simulink model "ex_blkCornerDetection_edited"  (R2023b)
settings: Solver=FixedStepDiscrete  StartTime=0.0  StopTime=0  RelTol=1e-3
undefined symbols (not defined in the file or in its folder): gray, Rec, SDTV
libraries: visiontextngfix x2, visionconversions x1, dspinverses x1, dspmathops x1, visionsources x1
settings Model: Creator=The MathWorks, Inc.  LastModifiedBy=Alyssa
settings DebuggingCC: ParameterPrecisionLossMsg=none  UnconnectedInputMsg=warning  UnconnectedOutputMsg=warning  UnconnectedLineMsg=warning  IntegerSaturationMsg=none
settings ModelReferenceCC: EnableRefExpFcnMdlSchedulingChecks=on
settings RTWCC: DLArmComputeVersion=19.05

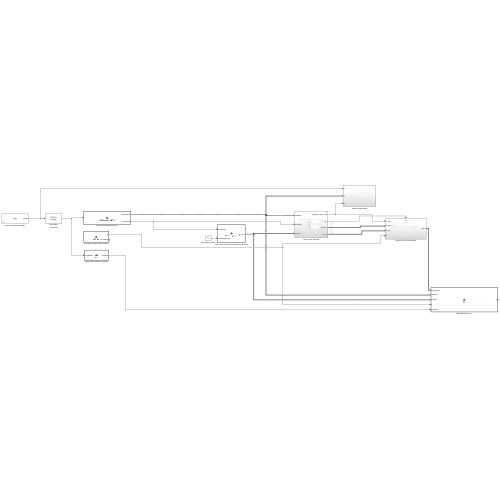
[thumbnail: Simulink's stored preview of the top-level diagram]
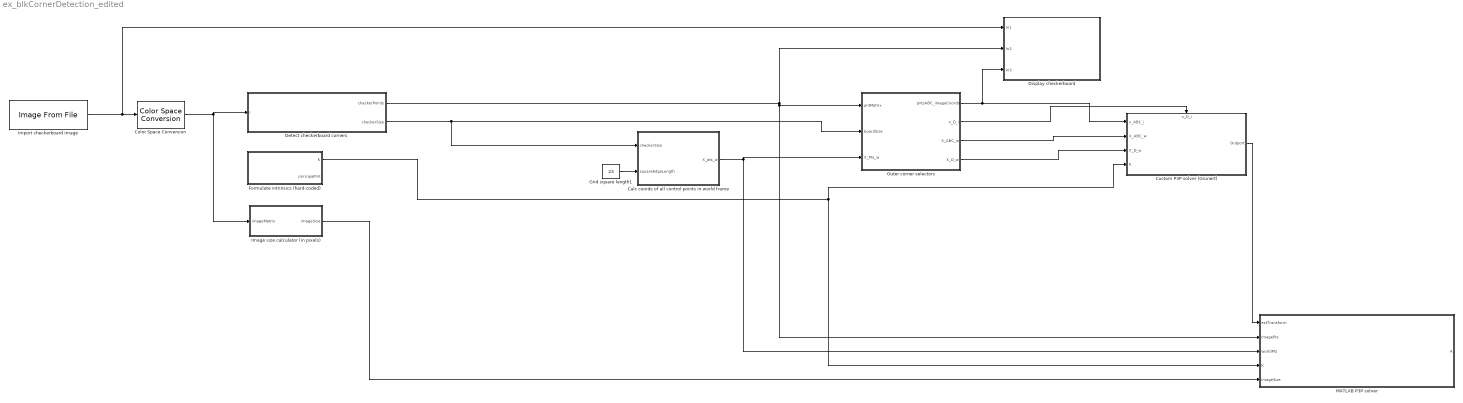
== system ex_blkCornerDetection_edited ==
  Calc coords of all control points in world frame : MATLAB Function  TreatAsAtomicUnit=on
  Color Space Conversion : visionconversions/Color Space  Conversion  conversion=Obsolete  conversionActive=R'G'B' to intensity  wp_str=D65  rec=Rec. 601 (SDTV)  sys=1125/60/2:1  imagePorts=One multidimensional signal
  Custom P3P solver (Grunert) : Subsystem
      settings: PortSchema="{\"entries\":[{\"content\":{\"sides\":[{\"content\":{\"connectorIds\":[\"In1\",\"In2\",\"In3\",\"In4\"]},\"type\":\"ConnectorPlacement.EquallySpacedRectSide\",\"uuid\":\"ab8d8f47-a078-4904-b229-676f132fd238\"},{\"content\":{\"connectorIds\":[\"Out1\"],\"side\":\"RIGHT\"},\"type\":\"ConnectorPlacement.EquallySpacedRectSide\",\"uuid\":\"00cb969a-2808-4efa-a104-ddec5f07b100\"},{\"content\":{\"connectorIds\":[\"In5\"],\"side\":\"TOP\"},\"type\":\"ConnectorPlacement.EquallySpacedRectSide\",\"uuid\":\"2fc50beb-0e06-41d1-87ca-520f8001ed43\"}]},\"type\":\"ConnectorPlacement.EquallySpacedConnector\",\"uuid\":\"61196fa6-a691-4b7f-8fee-5a47d7d03c1d\"}],\"packageUris\":[\"http://schema.mathworks.com/mf0/Connector/R2020b\"],\"version\":\"1.0\"}"
  Detect checkerboard corners : MATLAB Function  TreatAsAtomicUnit=on
  Display checkerboard : Subsystem
  Formulate intrinsics (hard-coded) : MATLAB Function  TreatAsAtomicUnit=on
  Grid square length1 : Constant  Value=23
  Image size calculator (in pixels) : MATLAB Function  TreatAsAtomicUnit=on
  Import checkerboard image : visionsources/Image From File  Tag=vipblks_nd  FileName=C:\Users\Alyssa\OneDrive - University of Cape Town\Vision\ESP32-CAM\CamCalibrationPics\8.jpg  Ts=inf  imagePorts=One multidimensional signal  OutPortLabels=R|G|B  ImageDataType=Inherit from input image  sdImageDataType=uint(8)  Signed=on  WordLength=16  FractionLengthMode=User-defined  FractionLength=15
  MATLAB P3P solver : MATLAB Function  TreatAsAtomicUnit=on
  Outer corner selectors : Subsystem
  wires:
  Color Space Conversion/1 -> Image size calculator (in pixels)/1(imageMatrix), Detect checkerboard corners/1(I)
  Import checkerboard image/1 -> Display checkerboard/1(In1), Color Space Conversion/1
  Detect checkerboard corners/2(checkerSize) -> Calc coords of all control points in world frame/1(checkerSize), Outer corner selectors/2(boardSize)
  Formulate intrinsics (hard-coded)/1(K) -> Custom P3P solver (Grunert)/4(K), MATLAB P3P solver/4(K)
  Custom P3P solver (Grunert)/1(Outport) -> MATLAB P3P solver/1(estTransform)
  Calc coords of all control points in world frame/1(X_pts_w) -> MATLAB P3P solver/3(worldPts), Outer corner selectors/3(X_Pts_w)
  Grid square length1/1 -> Calc coords of all control points in world frame/2(squareEdgeLength)
  Outer corner selectors/1(pntsABC_imageCoords) -> Custom P3P solver (Grunert)/1(x_ABC_i), Display checkerboard/3(In3)
  Outer corner selectors/2(x_D_i) -> Custom P3P solver (Grunert)/5(x_D_i)
  Outer corner selectors/3(X_ABC_w) -> Custom P3P solver (Grunert)/2(X_ABC_w)
  Outer corner selectors/4(X_D_w) -> Custom P3P solver (Grunert)/3(X_D_w)
  Detect checkerboard corners/1(checkerPoints) -> MATLAB P3P solver/2(imagePts), Outer corner selectors/1(pntMatrix), Display checkerboard/2(In2)
  Image size calculator (in pixels)/1(imageSize) -> MATLAB P3P solver/5(imageSize)

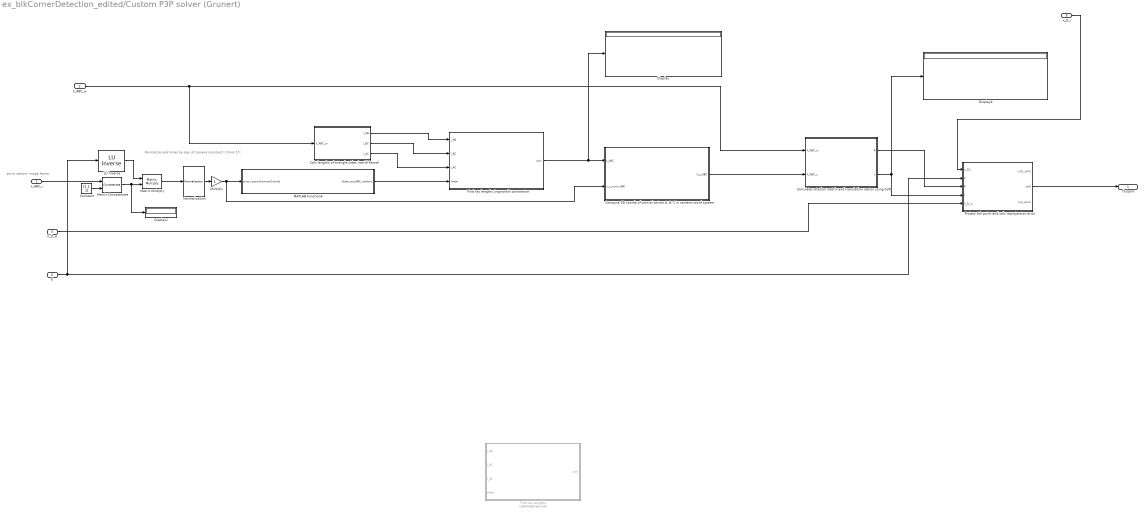
== system ex_blkCornerDetection_edited/Custom P3P solver (Grunert) ==
  note: point vectors image frame
  note: Normalize and times by sign of camera constant (I think 1?)
  x_ABC_i : Inport
  X_ABC_w : Inport  Port=2
  X_D_w : Inport  Port=3
  K : Inport  Port=4
  x_D_i : Inport  Port=5
  " LU Inverse" : dspinverses/ LU Inverse
  Calc lengths of triangle sides (world frame) : MATLAB Function  TreatAsAtomicUnit=on
  Calculate rotation matrix and translation vector using SVD : MATLAB Function  TreatAsAtomicUnit=on
  "Compute 3D coords of control points A, B, C in camera coord system" : MATLAB Function  TreatAsAtomicUnit=on
  Constant : Constant  Value=[1 1 1]  VectorParams1D=off
  Display : Display
  Display1 : Display
  Display4 : Display
  Find ray lengths : MATLAB Function  Commented=on  TreatAsAtomicUnit=on
  Find ray lengths jingnanshi convention : MATLAB Function  TreatAsAtomicUnit=on
  MATLAB Function4 : MATLAB Function  TreatAsAtomicUnit=on
  Matrix Concatenate : Concatenate  Mode=Multidimensional array
  Matrix Multiply : Product  Multiplication=Matrix(*)
  Multiply : Gain
  Normalization : dspmathops/Normalization  NormType=2-norm  Bias=1e-10  NormOver=Each column  Dimension=1  roundingMode=Floor  overflowMode=off  accumDataTypeStr=Inherit: Same as product output  accumLastDataTypeStr=Inherit: Same as product output  outputDataTypeStr=Inherit: Same as product output  outputMin=[]  outputMax=[]  outputLastDataTypeStr=Inherit: Same as product output
  Project 4th point and calc reprojection error : MATLAB Function  TreatAsAtomicUnit=on
  Outport : Outport
  wires:
  Calculate rotation matrix and translation vector using SVD/1(R) -> Project 4th point and calc reprojection error/3(R)
  Multiply/1 -> "Compute 3D coords of control points A, B, C in camera coord system"/2(x_c_norm_ABC), MATLAB Function4/1(pnts_vectorsCameraCoords)
  Normalization/1 -> Multiply/1
  MATLAB Function4/1(theta_raysABC_radians) -> Find ray lengths jingnanshi convention/4(theta)
  "Compute 3D coords of control points A, B, C in camera coord system"/1(X_c_ABC) -> Calculate rotation matrix and translation vector using SVD/2(X_ABC_c)
  Calculate rotation matrix and translation vector using SVD/2(t) -> Project 4th point and calc reprojection error/4(t), Display4/1
  X_D_w/1 -> Project 4th point and calc reprojection error/5(X_D_w)
  X_ABC_w/1 -> Calc lengths of triangle sides (world frame)/1(X_ABC_w), Calculate rotation matrix and translation vector using SVD/1(X_ABC_w)
  Calc lengths of triangle sides (world frame)/3(l_AC) -> Find ray lengths jingnanshi convention/3(l_AC)
  Calc lengths of triangle sides (world frame)/1(l_AB) -> Find ray lengths jingnanshi convention/1(l_AB)
  Calc lengths of triangle sides (world frame)/2(l_BC) -> Find ray lengths jingnanshi convention/2(l_BC)
  K/1 -> " LU Inverse"/1, Project 4th point and calc reprojection error/2(K)
  x_D_i/1 -> Project 4th point and calc reprojection error/1(x_D_i)
  Project 4th point and calc reprojection error/2(soln) -> Outport/1
  Find ray lengths jingnanshi convention/1(soln) -> "Compute 3D coords of control points A, B, C in camera coord system"/1(s_ABC), Display/1
  x_ABC_i/1 -> Matrix Concatenate/1
  Matrix Concatenate/1 -> Display1/1, Matrix Multiply/2
  " LU Inverse"/1 -> Matrix Multiply/1
  Matrix Multiply/1 -> Normalization/1
  Constant/1 -> Matrix Concatenate/2

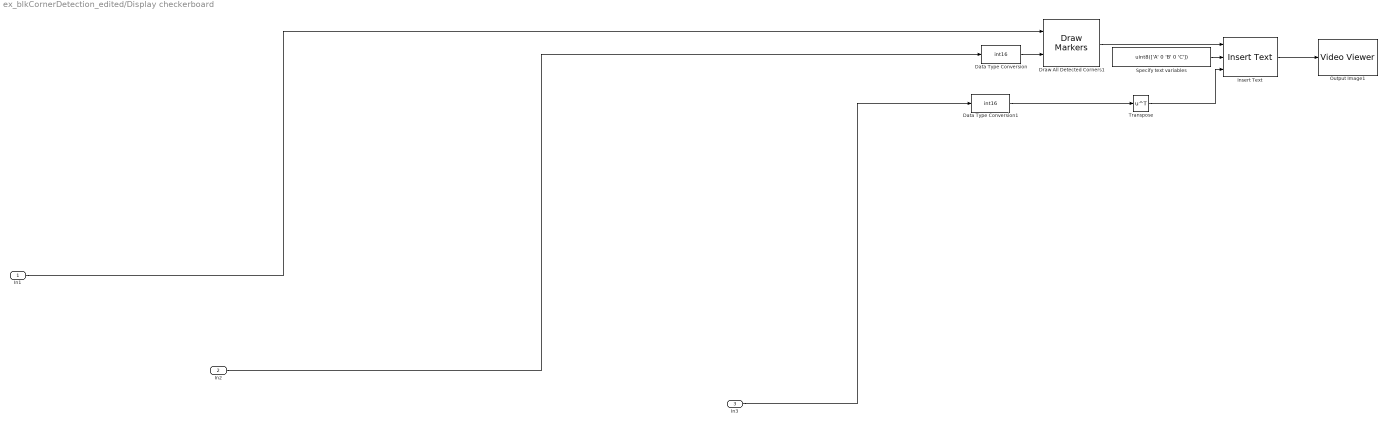
== system ex_blkCornerDetection_edited/Display checkerboard ==
  In1 : Inport
  In2 : Inport  Port=2
  In3 : Inport  Port=3
  Data Type Conversion : DataTypeConversion  OutDataTypeStr=int16  SaturateOnIntegerOverflow=off  RndMeth=Floor
  Data Type Conversion1 : DataTypeConversion  OutDataTypeStr=int16  SaturateOnIntegerOverflow=off  RndMeth=Floor
  Draw All Detected Corners1 : visiontextngfix/Draw Markers  shape=Circle  size=9  fill=on  fillClrSource=Specify via dialog  display=User-specified value  intensity=200  color=[250 0 0]  opacity=0.6  viewport=Entire image  antialiasing=off  inType=Obsolete  imagePorts=One multidimensional signal  roundingMode=Floor  overflowMode=off  memoryMode=Specify word length  memoryWordLength=16  memoryFracLength=15  prodOutputMode=Binary point scaling  prodOutputWordLength=32  prodOutputFracLength=14
  Insert Text : visiontextngfix/Insert Text  inputType=Obsolete  theText='%s'  getTextLocFrom=Input port  textLoc=[100 100]  getTextColorFrom=Specify via dialog  textColor=[0 255 0]  getTextIntensityFrom=Specify via dialog  textIntensity=1  getTextOpacityFrom=Specify via dialog  textOpacity=1.0  dummyVar2=0  dummyVar3=0  dummyVar4=0  imagePorts=One multidimensional signal  isInputTransposed=off  fontFace=LucidaSansRegular  dummyVar1=0  blockFontSize=60  antiAliased=on
  Output Image1 : VideoViewer  colormapValue=gray(256)  FigPos=[2113 930 833 715]
  Specify text variables : Constant  Value=uint8(['A' 0 'B' 0 'C'])
  Transpose : Math  Operator=transpose
  wires:
  Data Type Conversion/1 -> Draw All Detected Corners1/2
  Draw All Detected Corners1/1 -> Insert Text/1
  Specify text variables/1 -> Insert Text/2
  Transpose/1 -> Insert Text/3
  In1/1 -> Draw All Detected Corners1/1
  Insert Text/1 -> Output Image1/1
  Data Type Conversion1/1 -> Transpose/1
  In3/1 -> Data Type Conversion1/1
  In2/1 -> Data Type Conversion/1

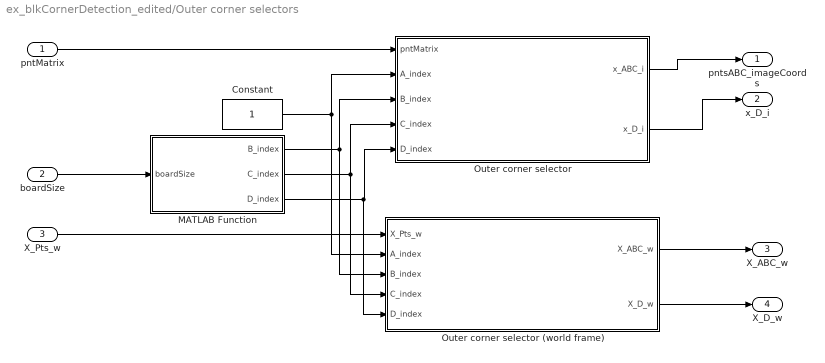
== system ex_blkCornerDetection_edited/Outer corner selectors ==
  pntMatrix : Inport
  boardSize : Inport  Port=2
  X_Pts_w : Inport  Port=3
  Constant : Constant
  MATLAB Function : MATLAB Function  TreatAsAtomicUnit=on
  Outer corner selector : MATLAB Function  TreatAsAtomicUnit=on
  Outer corner selector (world frame) : MATLAB Function  TreatAsAtomicUnit=on
  pntsABC_imageCoords : Outport
  x_D_i : Outport  Port=2
  X_ABC_w : Outport  Port=3
  X_D_w : Outport  Port=4
  wires:
  Outer corner selector/2(x_D_i) -> x_D_i/1
  Outer corner selector (world frame)/1(X_ABC_w) -> X_ABC_w/1
  Outer corner selector/1(x_ABC_i) -> pntsABC_imageCoords/1
  Outer corner selector (world frame)/2(X_D_w) -> X_D_w/1
  boardSize/1 -> MATLAB Function/1(boardSize)
  pntMatrix/1 -> Outer corner selector/1(pntMatrix)
  X_Pts_w/1 -> Outer corner selector (world frame)/1(X_Pts_w)
  Constant/1 -> Outer corner selector/2(A_index), Outer corner selector (world frame)/2(A_index)
  MATLAB Function/1(B_index) -> Outer corner selector/3(B_index), Outer corner selector (world frame)/3(B_index)
  MATLAB Function/2(C_index) -> Outer corner selector/4(C_index), Outer corner selector (world frame)/4(C_index)
  MATLAB Function/3(D_index) -> Outer corner selector (world frame)/5(D_index), Outer corner selector/5(D_index)

== matlab function ex_blkCornerDetection_edited/Custom P3P solver (Grunert)/Project 4th point and calc reprojection error ==
  data: x_D_i input; K input; R input; x_D_i_proj output size=[2,4]; t input; X_D_w input; soln output size=[3,4]; min_error output
function [x_D_i_proj, soln, min_error]= fcn(x_D_i, K, R, t, X_D_w)

%Calculate the projection of a fourth point onto the image plane, based on 
%the candidate rotation matrices and translation vectors. Later, we
%will check how well this corresponds with where it was actually observed.
    
    %Initialise vector
    x_D_i_proj = zeros(2,4); %where i stands for "image plane"
    x_D_i_proj_homo = zeros(3,4); %where i stands for "image plane"
    error = zeros(1,4);     %reprojection error
    soln = zeros(3, 4);

    %For each possible solution
    for n=1: size(R, 3)

        %Calculate projection of the point D
        x_D_i_proj_homo(:, n) = K * (  (R(:, :, n) * X_D_w)  + t(:,n)  );

        %Normalise by the 3rd dimension
        x_D_i_proj(1,n) = x_D_i_proj_homo(1,n)/x_D_i_proj_homo(3,n);
        x_D_i_proj(2,n) = x_D_i_proj_homo(2,n)/x_D_i_proj_homo(3,n);

        %Calculate reprojection error
        error(1, n) = norm(x_D_i - x_D_i_proj(:, n));
    
    end

    %Choose lower reprojection error
    error(1, 1) = norm(x_D_i - x_D_i_proj(:, 1));
    min_error = error(1,1);
    soln = [R(:, :, 1) t(:,1)];
    
    for j=2 : size(x_D_i_proj, 2)
        
        if error(1, j) < min_error
            min_error = error(1, j);
            soln = [R(:, :, j) t(:,j)]
        end
    
    end

== matlab function ex_blkCornerDetection_edited/MATLAB P3P solver ==
  data: estTransform input; imagePts input; worldPts input; K input; imageSize input; A output
function A = fcn(estTransform, imagePts, worldPts, K, imageSize)

    %imagePts_vert = transpose(imagePts);
    %worldPts_vert = transpose(worldPts);
    focalLngth = [K(1,1) K(2,2)];
    principalPnt = [K(1,3) K(2,3)];

    coder.extrinsic('builtinP3P');
    A = zeros(4,4);

    
    estTransform_R_inv = inv(estTransform(:, 1:3));
    estTransform_negTranslation_Rotated = estTransform_R_inv * (-estTransform(:, 4));

    A = builtinP3P(imagePts, worldPts, focalLngth, principalPnt, imageSize, estTransform_negTranslation_Rotated, estTransform_R_inv)

    %intr = cameraIntrinsics(focalLngth, principalPnt, imageSize)

    %worldPose = estworldpose(imagePts_vert, worldPts_vert, intr)

    %pcshow(worldPts,VerticalAxis="Y",VerticalAxisDir="down", ...
    %MarkerSize=30);
    %hold on
    %plotCamera(Size=10,Orientation=worldPose.R', ...
    %    Location=worldPose.Translation);
    %hold off

== matlab function ex_blkCornerDetection_edited/Image size calculator (in pixels) ==
  data: imageMatrix input; imageSize output
function imageSize = fcn(imageMatrix)

imageSize = [size(imageMatrix, 1) size(imageMatrix,2)];

== matlab function ex_blkCornerDetection_edited/Custom P3P solver (Grunert)/Find ray lengths jingnanshi convention ==
  data: l_AB input; soln output size=[4, 3]; l_BC input; l_AC input; theta input
function soln = fcn(l_AB, l_BC, l_AC, theta)

soln = zeros(4, 3);


%Calculate polynomial coefficients
a = l_AC;
b = l_BC;
c = l_AB;

gamma = theta(1); %theta_AB
alpha = theta(3); %theta_AC
beta = theta(2); %theta_BC


a2minc2ovb2 =  (a^2 - c^2) / b^2 ;
a2plusc2ovb2 =  (a^2 + c^2) / b^2; 


A0 = (1 + a2minc2ovb2)^2   -   4*((a*cos(gamma)/b)^2);
A1 = - a2minc2ovb2 * (1 + a2minc2ovb2) * cos(beta)     +    2 * ((a * cos(gamma) /  b)^2) * cos (beta)     -     (1 - a2plusc2ovb2) * cos(alpha) * cos(gamma);
A1 = 4 * A1;
A2 = a2minc2ovb2^2   -   1   +   2*((a2minc2ovb2 * cos(beta))^2)  +  2 *(  ((b^2 - c^2)/(b^2))  * (cos(alpha))^2  )   - 4*a2plusc2ovb2*cos(alpha)*cos(beta)*cos(gamma)   +   2*((b^2 - a^2)/(b^2))*((cos(gamma))^2);
A2 = 2* A2;
A3 = a2minc2ovb2 * (1 - a2minc2ovb2) * cos(beta)    -   (1 - a2plusc2ovb2) * cos(alpha) * cos(gamma)    +   2 * ((c * cos(alpha)/b)^2) * cos(beta);
A3 = 4 * A3;
A4 = (a2minc2ovb2 -1)^2   - (2 * c * cos(alpha) / b)^2;

%Solve polynomial
%instead of u and v for polynomial, use g and h - i.e., g = s2/s1 and h =
%s3/s1
p = [A4 A3 A2 A1 A0];
h = roots(p);
%choose only real roots - maybe this is not necessary?
h = h(imag(h)==0);
h = real(h);

%%%%%%%%%%%%%%%%%%%%%%%%%%%%%%%%%%%%%%%%%
%%%%%%%%%%%%%Find ray lengths

%For s1, which corresponds to sB. Should end up with 4 solns
%s_A =    (b^2) / (1 + h.^2  +  2*h*cos(beta)  )     ;
%s_A = s_A(s_A~=0);
%s_A = transpose(s_A);
%s_A = s_A.^0.5;


%Find s2, which corresponds to sC.
counter = 1
for i = 1:numel(h)

    s_1 = (b^2) / (1 + (h(i)^2) - 2*h(i)*cos(beta));
    s_1 = sqrt(s_1);

    G2 = s_1^2;
    G1 = - 2 * (s_1^2) * cos(gamma);
    G0 = (s_1^2 -c^2);

    g = roots([G2 G1 G0]);
    g = g(imag(g)==0);
    g = real(g);

    %First, solve for s_C, since it only depends on h and s_A:

    for j = 1:numel(g)
        soln(counter, 1) = s_1 * g(j);
        soln(counter, 3) = s_1 * h(i);
        soln(counter, 2) = s_1; 
        counter = counter +1
    end

end

== matlab function ex_blkCornerDetection_edited/Outer corner selectors/MATLAB Function ==
  data: boardSize input; B_index output; C_index output; D_index output
function [B_index, C_index, D_index]= fcn(boardSize)

B_index = boardSize(1) - 1;
C_index = ((boardSize(1) - 1) * (boardSize(2) - 2)) + 1;
D_index = ((boardSize(1) - 1) * (boardSize(2) - 1)) ;

== matlab function ex_blkCornerDetection_edited/Calc coords of all control points in world frame ==
  data: X_pts_w output size=[60, 3]; checkerSize input; squareEdgeLength input
function X_pts_w = calcPtoPLengths_world(checkerSize, squareEdgeLength)
    
    boardWidth = checkerSize(2);
    boardHeight = checkerSize(1);
    X_pts_w = zeros((boardWidth-1)*(boardHeight-1), 3)

    %for each column
    for c=1 : boardWidth-1
        for r = 1: boardHeight-1
            x = (c-1)*squareEdgeLength;
            y = (r-1)*squareEdgeLength;
            z = 0;
            X_pts_w(  (((c-1)*(boardHeight-1)) + r), 1) = x;
            X_pts_w(  (((c-1)*(boardHeight-1)) + r), 2) = y;
            X_pts_w(  (((c-1)*(boardHeight-1)) + r), 3) = z;
        end
    end

== matlab function ex_blkCornerDetection_edited/Custom P3P solver (Grunert)/Calc lengths of triangle sides (world frame) ==
  data: X_ABC_w input; l_AB output; l_BC output; l_AC output
function [l_AB, l_BC, l_AC]= fcn(X_ABC_w)

l_AB = norm(X_ABC_w(:,1)-X_ABC_w(:,2));
l_AC = norm(X_ABC_w(:,1)-X_ABC_w(:,3));
l_BC = norm(X_ABC_w(:,2)-X_ABC_w(:,3));

== matlab function ex_blkCornerDetection_edited/Detect checkerboard corners ==
  data: checkerPoints output size=[60, 2]; I input; checkerSize output size=[1, 2]
function [checkerPoints, checkerSize]= findCheckerboardPnts(I)

%I = imread(fullfile('C:\Users\Alyssa\OneDrive - University of Cape Town\Vision\ESP32-CAM\CamCalibrationPics', '1.jpg'));
Points = detectCheckerboardPoints(I);
[~,checkerSize] = detectCheckerboardPoints(I)
checkerPoints = round(Points);
%checkerSize = Size;
%checkerPoints = imagePoints;

== matlab function ex_blkCornerDetection_edited/Formulate intrinsics (hard-coded) ==
  data: K output; principalPnt output
function [K, principalPnt]= intrinsics

    fx = 1274.58238813250;
    fy = 1273.36371905619;
    Ox = 627.693937913345;
    Oy = 405.441250468717;

    K = [fx 0 Ox; 0 fy Oy; 0 0 1];

    principalPnt = [627.693937913345; 405.441250468717];

== matlab function ex_blkCornerDetection_edited/Outer corner selectors/Outer corner selector (world frame) ==
  data: X_Pts_w input; X_ABC_w output size=[3, 3]; X_D_w output size=[3, 1]; A_index input; B_index input; C_index input; D_index input
function [X_ABC_w, X_D_w]= calcPtoPLengths_world(X_Pts_w, A_index, B_index, C_index, D_index)
    
    X_A_w = X_Pts_w(A_index, :);
    X_B_w = X_Pts_w(B_index, :);
    X_C_w = X_Pts_w(C_index, :);
    X_D_w_vert = X_Pts_w(D_index, :);

    X_ABC_w_vert = [X_A_w; X_B_w; X_C_w];
    X_ABC_w = transpose(X_ABC_w_vert);
    X_D_w = transpose(X_D_w_vert);

== matlab function ex_blkCornerDetection_edited/Outer corner selectors/Outer corner selector ==
  data: x_ABC_i output; x_D_i output; pntMatrix input; A_index input; B_index input; C_index input; D_index input
function [x_ABC_i, x_D_i] = calcPntVectors_PrincipalPntToImagePlane(pntMatrix, A_index, B_index, C_index, D_index)

%Obtain pixel positions
A_u = pntMatrix(A_index,1);
A_v = pntMatrix(A_index,2);

B_u = pntMatrix(B_index, 1);
B_v = pntMatrix(B_index, 2);

C_u = pntMatrix( C_index , 1);
C_v = pntMatrix( C_index , 2);

D_u = pntMatrix( D_index, 1);
D_v = pntMatrix(D_index, 2);


%Created augmented U matrices - i.e., add extra row of "1"
x_ABC_i = [A_u B_u C_u; A_v B_v C_v]
%pnts_U_ABC_aug = [pnts_U_ABC; 1 1 1];

%pnts_X_c = inv(K) * pnts_U_ABC_aug;

%pntVectors_cameraCoords = pnts_X_c;
%pntsABC_imageCoords = pnts_U_ABC;
%pntsABCD_imageCoords = [A_u B_u C_u D_u; A_v B_v C_v D_v];
x_D_i = [D_u; D_v];

== matlab function ex_blkCornerDetection_edited/Custom P3P solver (Grunert)/MATLAB Function4 ==
  data: pnts_vectorsCameraCoords input; theta_raysABC_radians output
function theta_raysABC_radians = calcProjectionRayAngles(pnts_vectorsCameraCoords)

A_x_c = pnts_vectorsCameraCoords(:,1);
B_x_c = pnts_vectorsCameraCoords(:,2);
C_x_c = pnts_vectorsCameraCoords(:,3);

%theta_AB = acos(dot(A_x_c, B_x_c));
%theta_BC = acos(dot(B_x_c, C_x_c));
%theta_AC = acos(dot(C_x_c, A_x_c));

%theta_AB = atan2(norm(cross(A_x_c, B_x_c)), dot(A_x_c, B_x_c));
%theta_BC = atan2(norm(cross(B_x_c, C_x_c)), dot(B_x_c, C_x_c));
%theta_AC = atan2(norm(cross(A_x_c, C_x_c)), dot(A_x_c, C_x_c)); 

theta_AB = acos(dot(A_x_c, B_x_c)/(norm(A_x_c)*norm(B_x_c)));
theta_BC = acos(dot(B_x_c, C_x_c)/(norm(B_x_c)*norm(C_x_c)));
theta_AC = acos(dot(A_x_c, C_x_c)/(norm(A_x_c)*norm(C_x_c)));


theta_raysABC_radians = [theta_AB; theta_BC; theta_AC];

== matlab function ex_blkCornerDetection_edited/Custom P3P solver (Grunert)/Find ray lengths ==
  data: l_AB input; soln output size=[4, 3]; l_BC input; l_AC input; theta input
function soln = fcn(l_AB, l_BC, l_AC, theta)

soln = zeros(4, 3);


%Calculate polynomial coefficients
a = l_BC;
b = l_AC;
c = l_AB;

gamma = theta(3); %theta_AC
alpha = theta(2); %theta_BC
beta = theta(1); %theta_AB


a2minc2ovb2 =  (a^2 - c^2) / b^2 ;
a2plusc2ovb2 =  (a^2 + c^2) / b^2; 


A0 = (1 + a2minc2ovb2)^2   -   4*((a*cos(gamma)/b)^2);
A1 = - a2minc2ovb2 * (1 + a2minc2ovb2) * cos(beta)     +    2 * ((a * cos(gamma) /  b)^2) * cos (beta)     -     (1 - a2plusc2ovb2) * cos(alpha) * cos(gamma);
A1 = 4 * A1;
A2 = a2minc2ovb2^2   -   1   +   2*((a2minc2ovb2 * cos(beta))^2)  +  2 *(  ((b^2 - c^2)/(b^2))  * (cos(alpha))^2  )   - 4*a2plusc2ovb2*cos(alpha)*cos(beta)*cos(gamma)   +   2*((b^2 - a^2)/(b^2))*(cos(gamma)^2);
A2 = 2* A2;
A3 = a2minc2ovb2 * (1 - a2minc2ovb2) * cos(beta)    -   (1 - a2plusc2ovb2) * cos(alpha) * cos(gamma)    +   2 * ((c * cos(alpha)/b)^2) * cos(beta);
A3 = 4 * A3;
A4 = (a2minc2ovb2 -1)^2   - (2 * c * cos(alpha) / b)^2;

%Solve polynomial
%instead of u and v for polynomial, use g and h - i.e., g = s2/s1 and h =
%s3/s1
p = [A4 A3 A2 A1 A0];
h = roots(p);
%choose only real roots - maybe this is not necessary?
h = h(imag(h)==0);
h = real(h);

%%%%%%%%%%%%%%%%%%%%%%%%%%%%%%%%%%%%%%%%%
%%%%%%%%%%%%%Find ray lengths

%For s1, which corresponds to sA. Should end up with 4 solns
%s_A =    (b^2) / (1 + h.^2  +  2*h*cos(beta)  )     ;
%s_A = s_A(s_A~=0);
%s_A = transpose(s_A);
%s_A = s_A.^0.5;


%Find s2, which corresponds to sC.
counter = 1
for i = 1:numel(h)

    s_A = (b^2) / (1 + (h(i)^2) - 2*h(i)*cos(beta));
    s_A = sqrt(s_A);

    G2 = s_A^2;
    G1 = - 2 * (s_A^2) * cos(gamma);
    G0 = (s_A -c)^2;

    g = roots([G2 G1 G0]);
    g = g(imag(g)==0);
    g = real(g);

    %First, solve for s_C, since it only depends on h and s_A:

    for j = 1:numel(g)
        soln(counter, 1) = s_A;
        soln(counter, 3) = s_A * g(j);
        soln(counter, 2) = h(i) * s_A;
        counter = counter +1
    end

end

== matlab function ex_blkCornerDetection_edited/Custom P3P solver (Grunert)/Compute 3D coords of control points A, B, C in camera coord system ==
  data: s_ABC input; X_c_ABC output size=[3,3,4]; x_c_norm_ABC input
function X_c_ABC = fcn(s_ABC, x_c_norm_ABC)
    X_c_ABC = zeros(3,3,4);


    %For each combination of possible lengths
    for n=1:size(s_ABC, 1)
        %Get the vector between the camera and the point by multiplying
        %each element of the (unit) direction vector with the associated
        %ray length from the solution. 
        %The solution takes the form: [s_A1 s_B1 s_C1; s_A2 sB2...].
        %The direction vectors take the form: [xA xB xC; yA yB...].
        X_c_ABC(:, 1, n) = s_ABC(n, 1) * x_c_norm_ABC(:, 1);
        X_c_ABC(:, 2, n) = s_ABC(n, 2) * x_c_norm_ABC(:, 2);
        X_c_ABC(:, 3, n) = s_ABC(n, 3) * x_c_norm_ABC(:, 3);
    end

== matlab function ex_blkCornerDetection_edited/Custom P3P solver (Grunert)/Calculate rotation matrix and translation vector using SVD ==
  data: X_ABC_w input; R output size=[3,3,4]; X_ABC_c input; t output size=[3,4]
function [R, t]= fcn(X_ABC_w, X_ABC_c)

%We have 3 points in the world frame and in the camera frame. Now we need 
%to find the rotation and translation matrices that would convert one to 
%the other.
%This is the classic Procrustes problem, which we can solve using singular 
%value decomposition. We will end up with one rotation matrix and one
%translation vector for each of the possible sets of coordinates. 

 R = zeros(3,3,4);
 t = zeros(3,4);

 P = X_ABC_w;
 %Find the mean of the columns (i.e. the centroid of the shape)
 P_centroid = mean(P,2);
 %Centre each vector
 Q = P - P_centroid;

%for each possible solution
for i=1: size(X_ABC_c, 3)

    %Condition each vector as above
    P_dash =  X_ABC_c(:, :, i);
    P_dash_centroid = mean(P_dash, 2);
    Q_dash = P_dash - P_dash_centroid;
    
    %Find the covariance matrix
    H = Q_dash * transpose(Q);

    %Perform SVD (singular value decomposition)
    [U, S, V] = svd(H);

    %Calculate rotation matrix
    R(:,:,i) = U * transpose(V);
    %Correct sign if needed
    if det(R(:,:,i))<0
        U(:,end) = U(:,end) * (-1);
        %and recompute R
        R(:, :, i) = U * transpose(V);
    end

    %Calculate the translation vector:
    t(:, i) = P_dash_centroid - R(:, :, i)*P_centroid

end
